simulink library "DYN_AERO"  (Simulink 10.1)
settings: Solver=VariableStepAuto  StartTime=0.0  StopTime=10.0  RelTol=1e-3
undefined symbols (not defined in the file): DYN_AERO_par, IAU
libraries: vrlib x1, aerolibtransform2 x1, aerolibatmos2 x1
settings Model: Creator=Mahal  LastModifiedBy=m_mam

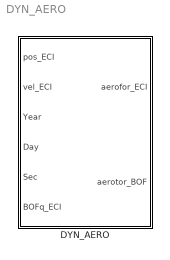
== system DYN_AERO ==
  DYN_AERO : Subsystem

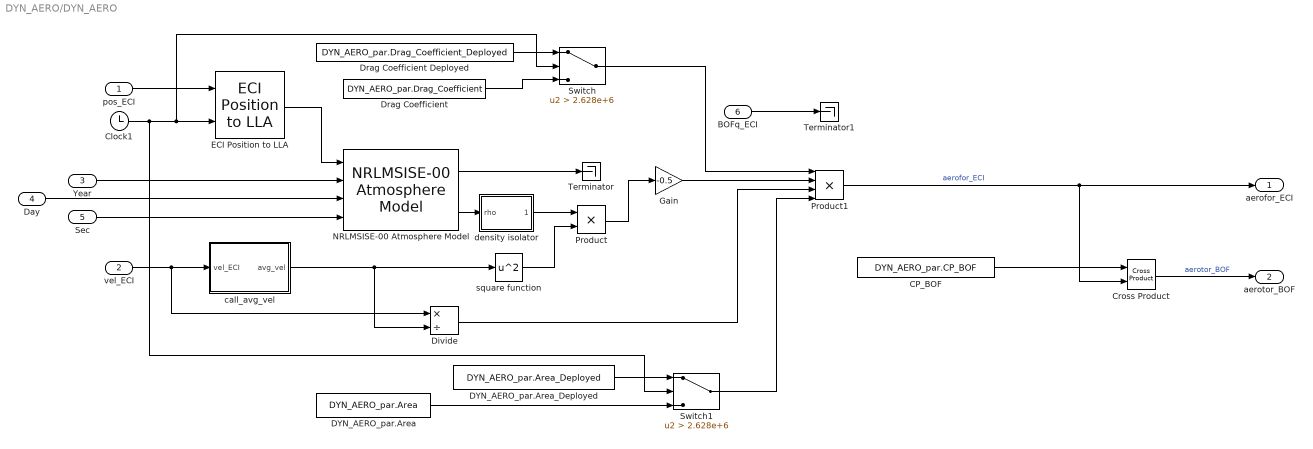
== system DYN_AERO/DYN_AERO ==
  pos_ECI : Inport
  "vel_ECI " : Inport  Port=2
  Year : Inport  Port=3
  Day : Inport  Port=4
  "Sec " : Inport  Port=5
  BOFq_ECI : Inport  Port=6
  CP_BOF : Constant  Value=DYN_AERO_par.CP_BOF
  Clock1 : Clock
  Cross Product : vrlib/Utilities/Cross Product
  DYN_AERO_par.Area : Constant  Value=DYN_AERO_par.Area
  DYN_AERO_par.Area_Deployed : Constant  Value=DYN_AERO_par.Area_Deployed
  Divide : Product  Inputs=*/
  "Drag Coefficient " : Constant  Value=DYN_AERO_par.Drag_Coefficient
  Drag Coefficient Deployed : Constant  Value=DYN_AERO_par.Drag_Coefficient_Deployed
  ECI Position to LLA : aerolibtransform2/ECI Position to LLA  red=IAU-2000/2006  year=2018  month=January  day=1  hour=0  min=0  sec=0  deltaT=Sec  errorflag=Error  extraparamflag=off  eunits=Metric (MKS)  earthmodel=WGS84  flat=1/298.257223563  eqradius=6378137
      settings: AttributesFormatString=%<red>  SourceProductBaseCode=AE
  Gain : Gain  Gain=-0.5
  NRLMSISE-00 Atmosphere Model : aerolibatmos2/NRLMSISE-00 Atmosphere Model  units=Metric (MKS)  lst_input=off  flux_ap_input=off  flags_input=Internal  flags=ones(1,23)  oxygen_in=on  action=Warning
      settings: SourceProductBaseCode=AE
  Product : Product
  Product1 : Product  Inputs=4
  Switch : Switch  Criteria=u2 > Threshold  Threshold=2.628e+6
  Switch1 : Switch  Criteria=u2 > Threshold  Threshold=2.628e+6
  Terminator : Terminator
  Terminator1 : Terminator
  call_avg_vel : MATLAB Function  TreatAsAtomicUnit=on
  density isolator : MATLAB Function  TreatAsAtomicUnit=on
  square function : Math  Operator=square  SignedPower=on  OutputSignalType=real  SaturateOnIntegerOverflow=on
  aerofor_ECI : Outport  VectorParamsAs1DForOutWhenUnconnected=off
  aerotor_BOF : Outport  Port=2  VectorParamsAs1DForOutWhenUnconnected=off
  wires:
  square function/1 -> Product/2
  Day/1 -> NRLMSISE-00 Atmosphere Model/3
  Year/1 -> NRLMSISE-00 Atmosphere Model/2
  Product/1 -> Gain/1
  "Sec "/1 -> NRLMSISE-00 Atmosphere Model/4
  NRLMSISE-00 Atmosphere Model/1 -> Terminator/1
  ECI Position to LLA/1 -> NRLMSISE-00 Atmosphere Model/1
  pos_ECI/1 -> ECI Position to LLA/1
  NRLMSISE-00 Atmosphere Model/2 -> density isolator/1(rho)
  density isolator/1(rho_avg) -> Product/1
  BOFq_ECI/1 -> Terminator1/1
  call_avg_vel/1(avg_vel) -> Divide/2, square function/1
  Clock1/1 -> Switch1/2, Switch/2, ECI Position to LLA/2
  Cross Product/1 -> aerotor_BOF/1  "aerotor_BOF"
  Drag Coefficient Deployed/1 -> Switch/1
  "Drag Coefficient "/1 -> Switch/3
  Switch/1 -> Product1/1
  Gain/1 -> Product1/2
  DYN_AERO_par.Area/1 -> Switch1/3
  Product1/1 -> Cross Product/2, aerofor_ECI/1  "aerofor_ECI"
  "vel_ECI "/1 -> Divide/1, call_avg_vel/1(vel_ECI)
  Divide/1 -> Product1/3
  CP_BOF/1 -> Cross Product/1
  DYN_AERO_par.Area_Deployed/1 -> Switch1/1
  Switch1/1 -> Product1/4

== matlab function DYN_AERO/call_avg_vel ==
  data: vel_ECI input double; avg_vel output double
function avg_vel = call_avg_vel(vel_ECI)

avg_vel = sqrt(vel_ECI(1)^2+vel_ECI(2)^2+vel_ECI(3)^2);

end

== matlab function DYN_AERO/density isolator ==
  data: rho input double; rho_avg output double
function rho_avg = density(rho)

rho_avg = rho(6);
